simulink model "test_master_task"  (Simulink 3.00)
libraries: mathlib x6, inoutlib x2, genlib x1, arclib x1

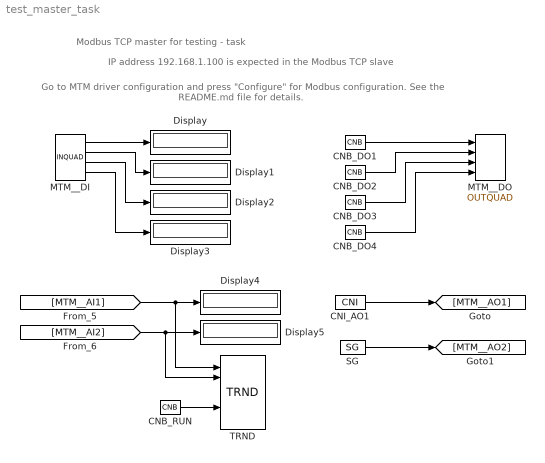
== system test_master_task ==
  note: IP address 192.168.1.100 is expected in the Modbus TCP slave
  note: Go to MTM driver configuration and press "Configure" for Modbus configuration.
      |
      | See the README.md file for details.
  note: Modbus TCP master for testing - task
  CNB_DO1 : mathlib/CNB  YCN=off
  CNB_DO2 : mathlib/CNB  YCN=on
  CNB_DO3 : mathlib/CNB  YCN=off
  CNB_DO4 : mathlib/CNB  YCN=on
  CNB_RUN : mathlib/CNB  YCN=on
  CNI_AO1 : mathlib/CNI  icn=2047
  Display{,1..5} (6 alike) : Display
      settings: Format=Best fit
  MTM__DI : inoutlib/INQUAD
  MTM__DO : inoutlib/OUTQUAD
  SG : genlib/SG  isig=1: SINE  amp=2047  freq=0.1  phase=0  offset=2047  ifrunit=1: Hz  iphunit=1: degrees
  TRND : arclib/TRND  n=4  l=1000  btype=8: Double  ptype1=1: Store  ptype2=1: Store  ptype3=1: Store  ptype4=1: Store  pfac=1  afac=0  arc=0  id=1  Title=Trend Title  timesrc=1
  wires:
  CNB_DO1/1 -> MTM__DO/1
  CNB_DO2/1 -> MTM__DO/2
  CNB_DO3/1 -> MTM__DO/3
  CNB_DO4/1 -> MTM__DO/4
  CNB_RUN/1 -> TRND/5
  CNI_AO1/1 -> [MTM__AO1]
  [MTM__AI1] -> Display4/1, TRND/1
  [MTM__AI2] -> Display5/1, TRND/2
  MTM__DI/1 -> Display/1
  MTM__DI/2 -> Display1/1
  MTM__DI/3 -> Display2/1
  MTM__DI/4 -> Display3/1
  SG/1 -> [MTM__AO2]
